simulink model "electrolizador"  (R2021a)
settings: Solver=VariableStepAuto  StartTime=0.0  StopTime=inf  RelTol=1e-3
undefined symbols (not defined in the file): magnitude
libraries: spspowerguiLib x1
settings Model: Creator=Usuario  LastModifiedBy=Usuario

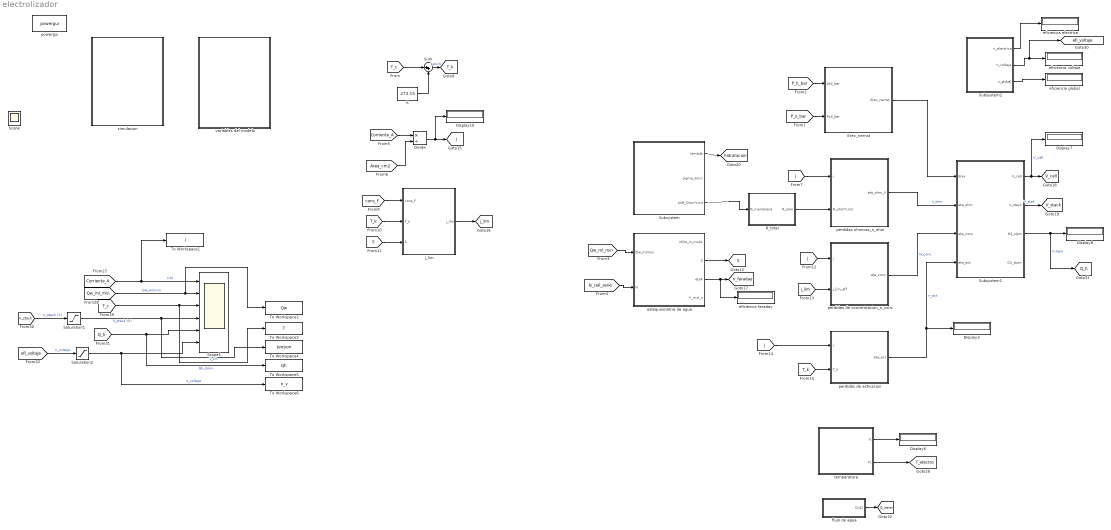
== system electrolizador ==
  Display{3,6..8,10} (5 alike) : Display
  Divide : Product  Inputs=*/
  Erev_nernst : Subsystem
  K : Constant  Value=273.15
  R_total : Subsystem
  Saturation1 : Saturate  UpperLimit=3  LowerLimit=0
  Saturation2 : Saturate  UpperLimit=1.1  LowerLimit=0
  Scope : Scope
  Scope1 : Scope  NumInputPorts=6
  Subsystem : Subsystem
  Subsystem1 : Subsystem
  Subsystem2 : Subsystem
  Sum : Sum  Inputs=|++
  To Workspace1 : ToWorkspace  VariableName=I  SaveFormat=Timeseries  SampleTime=-1
  To Workspace2 : ToWorkspace  VariableName=Qw  SaveFormat=Timeseries  SampleTime=-1
  To Workspace3 : ToWorkspace  VariableName=T  SaveFormat=Timeseries  SampleTime=-1
  To Workspace4 : ToWorkspace  VariableName=tension  SaveFormat=Timeseries  SampleTime=-1
  To Workspace5 : ToWorkspace  VariableName=Qh  SaveFormat=Timeseries  SampleTime=-1
  To Workspace6 : ToWorkspace  VariableName=n_v  SaveFormat=Timeseries  SampleTime=-1
  eficiencia electrica : Display
  eficiencia faraday : Display
  eficiencia global : Display
  eficiencia voltaje : Display
  estequiometria de agua : Subsystem
  flujo de agua : Subsystem
  j_lim : Subsystem
  perdidas de activacion : Subsystem
  perdidas de concentracion_n_conc : Subsystem
  perdidas ohmicas_n_ohm : Subsystem
  powergui : spspowerguiLib/powergui  Priority=1  SimulationMode=Discrete  SampleTime=50e-6  frequency=60  Iterations=50  frequencyindice=60  Pbase=100e6  ErrMax=1e-4  UnitsV=kV  UnitsW=MW  buscounter=0  FunctionMessages=off  echomessages=off  EnableUseOfTLC=off  CurrentSourceSwitches=off  DisableSnubberDevices=off  DisableRonSwitches=off  DisableVfSwitches=off  DisplayEquations=off  AutomaticDiscreteSolvers=off  SolverType=Tustin/Backward Euler (TBE)  Interpol=off  ExternalGateDelay=off  methode=off  Ts=100  x0status=blocks  SPID=on  SwTol=0  HookPort=off  NonlinearTolerance=1e-4  nMaxIteration=100  ContinueOnMaxIteration=off  RestoreLinks=warning  ResistiveCurrentMeasurement=off  Frange=[0:2:500]  Ylog=off  Xlog=on  ShowGrid=off  save=off  variable=ZData  structure=0  ZoomFFT=off  StartTime=0.0  cycles=1  DisplayStyle=1  fundamental=60  FreqAxis=off  MaxFrequency=1000  frequencyindicesteady=1  RmsSteady=1  display=off
  simulacion : Subsystem
  temperatura : Subsystem
  variables del modelo : Subsystem
  tag scope: Q_h=global, Q_water=global, S=global, T_electro=global, T_k=global, V_cell=global, V_stack=global, efi_voltaje=global, hidratacion=global, j=global, j_lim=global, n_faraday=global
  wires:
  K/1 -> Sum/2
  [T_c] -> Sum/1
  Sum/1 -> [T_k]  "kelvin"
  [P_o_bar] -> Erev_nernst/2(Po2_bar)
  [P_h_bar] -> Erev_nernst/1(ph2_bar)
  [Qw_ml_min] -> estequiometria de agua/1(Qw_ml/min)
  [N_cell_serie] -> estequiometria de agua/2(N)
  estequiometria de agua/2(S) -> [S]
  [Corriente_A] -> Divide/1
  [Area_cm2] -> Divide/2
  Divide/1 -> Display10/1, [j]
  Subsystem/3(ASR_Ohm*cm2) -> R_total/1(R_membrana)
  R_total/1(R_ohm) -> perdidas ohmicas_n_ohm/2(R_ohm*cm2)
  [j] -> perdidas ohmicas_n_ohm/1(j)
  [cons_F] -> j_lim/1(cons_F)
  [S] -> j_lim/3(S)
  [T_k] -> j_lim/2(T_k)
  j_lim/1(j_lim) -> [j_lim]
  [j] -> perdidas de concentracion_n_conc/1(j)
  [j_lim] -> perdidas de concentracion_n_conc/2(j_lim_eff)
  [T_k] -> perdidas de activacion/2(T_k)
  Erev_nernst/1(Erev_nernst) -> Subsystem1/1(Erev)
  perdidas ohmicas_n_ohm/1(eta_ohm_V) -> Subsystem1/2(eta_ohm)  "n_ohm"
  perdidas de concentracion_n_conc/1(eta_conc) -> Subsystem1/3(eta_conc)  "N_conc"
  estequiometria de agua/3(etaF) -> eficiencia faraday/1, [n_faraday]
  perdidas de activacion/1(eta_act) -> Subsystem1/4(eta_act), Display3/1  "n_act"
  Subsystem1/1(V_cell) -> Display7/1, [V_cell]  "V_cell"
  Subsystem1/2(V_stack) -> [V_stack]  "V_stak"
  Subsystem1/3(H2_slpm) -> [Q_h], Display8/1  "h slpm"
  Subsystem2/2(n_voltaje) -> [efi_voltaje], eficiencia voltaje/1
  Subsystem2/3(n_global) -> eficiencia global/1
  Subsystem/1(lambda) -> [hidratacion]
  [j] -> perdidas de activacion/1(j)
  temperatura/1(K) -> Display6/1
  temperatura/2(ºc) -> [T_electro]
  Subsystem2/1(n_electrica) -> eficiencia electrica/1
  [Corriente_A] -> To Workspace1/1, Scope1/1  "I(A)"
  [Qw_ml_min] -> To Workspace2/1, Scope1/2  "Qw_ml/min"
  [T_c] -> To Workspace3/1, Scope1/3  "T_Cº"
  [V_stack] -> Saturation1/1  "V_stack (V)"
  [Q_h] -> To Workspace5/1, Scope1/5  "Qh_l/min"
  [efi_voltaje] -> Saturation2/1  "n_voltaje"
  Saturation1/1 -> To Workspace4/1, Scope1/4  "V_stack (V)"
  Saturation2/1 -> To Workspace6/1, Scope1/6  "n_voltaje"
  flujo de agua/1(Out1) -> [Q_water]

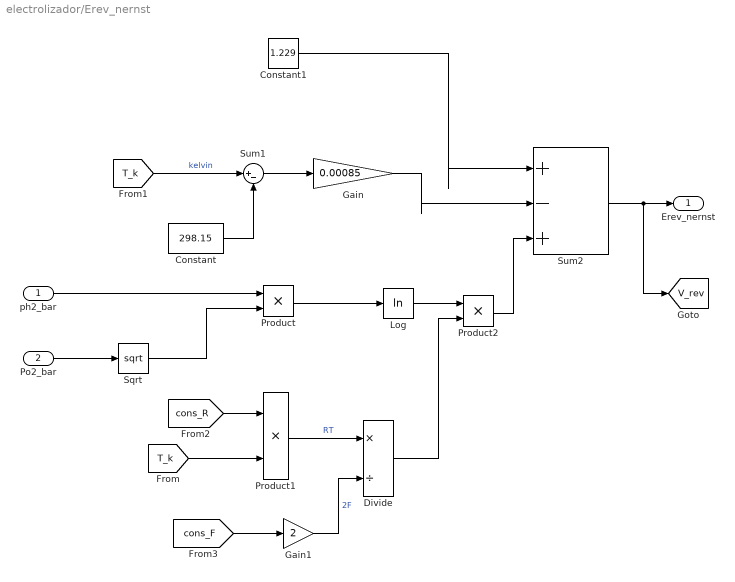
== system electrolizador/Erev_nernst ==
  ph2_bar : Inport
  Po2_bar : Inport  Port=2
  Constant : Constant  Value=298.15
  Constant1 : Constant  Value=1.229
  Divide : Product  Inputs=*/
  Gain : Gain  Gain=0.00085
  Gain1 : Gain  Gain=2
  Log : Math  Operator=log  SaturateOnIntegerOverflow=on
  Product : Product
  Product1 : Product
  Product2 : Product
  Sqrt : Sqrt  SaturateOnIntegerOverflow=on
  Sum1 : Sum  Inputs=|+-
  Sum2 : Sum  Inputs=|+-+
  Erev_nernst : Outport
  tag scope: V_rev=global
  wires:
  [T_k] -> Sum1/1  "kelvin"
  Constant/1 -> Sum1/2
  Sum1/1 -> Gain/1
  Po2_bar/1 -> Sqrt/1
  ph2_bar/1 -> Product/1
  Sqrt/1 -> Product/2
  Constant1/1 -> Sum2/1
  Gain/1 -> Sum2/2
  Product/1 -> Log/1
  [T_k] -> Product1/2
  [cons_R] -> Product1/1
  Product1/1 -> Divide/1  "RT"
  [cons_F] -> Gain1/1
  Gain1/1 -> Divide/2  "2F"
  Log/1 -> Product2/1
  Divide/1 -> Product2/2
  Product2/1 -> Sum2/3
  Sum2/1 -> [V_rev], Erev_nernst/1

== system electrolizador/R_total ==
  R_membrana : Inport
  Sum : Sum  Inputs=|++
  R_ohm : Outport
  wires:
  Sum/1 -> R_ohm/1
  R_membrana/1 -> Sum/1
  [R_contacto] -> Sum/2

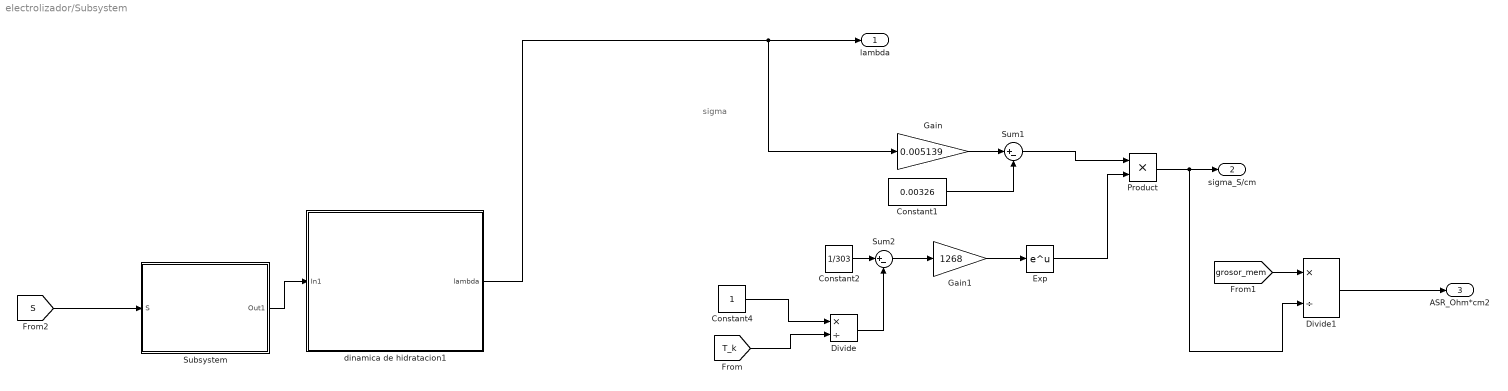
== system electrolizador/Subsystem ==
  note: sigma
  Constant1 : Constant  Value=0.00326
  Constant2 : Constant  Value=1/303
  Constant4 : Constant
  Divide : Product  Inputs=*/
  Divide1 : Product  Inputs=*/
  Exp : Math  SaturateOnIntegerOverflow=on
  Gain : Gain  Gain=0.005139
  Gain1 : Gain  Gain=1268
  Product : Product
  Subsystem : Subsystem
  Sum1 : Sum  Inputs=|+-
  Sum2 : Sum  Inputs=|+-
  dinamica de hidratacion1 : Subsystem
  lambda : Outport
  sigma_S/cm : Outport  Port=2
  ASR_Ohm*cm2 : Outport  Port=3
  wires:
  [grosor_mem] -> Divide1/1
  [T_k] -> Divide/2
  Sum2/1 -> Gain1/1
  Exp/1 -> Product/2
  Divide/1 -> Sum2/2
  Constant1/1 -> Sum1/2
  Gain/1 -> Sum1/1
  Gain1/1 -> Exp/1
  Constant4/1 -> Divide/1
  Constant2/1 -> Sum2/1
  Sum1/1 -> Product/1
  dinamica de hidratacion1/1(lambda) -> Gain/1, lambda/1
  Subsystem/1(Out1) -> dinamica de hidratacion1/1(In1)
  [S] -> Subsystem/1(S)
  Divide1/1 -> ASR_Ohm*cm2/1
  Product/1 -> Divide1/2, sigma_S/cm/1

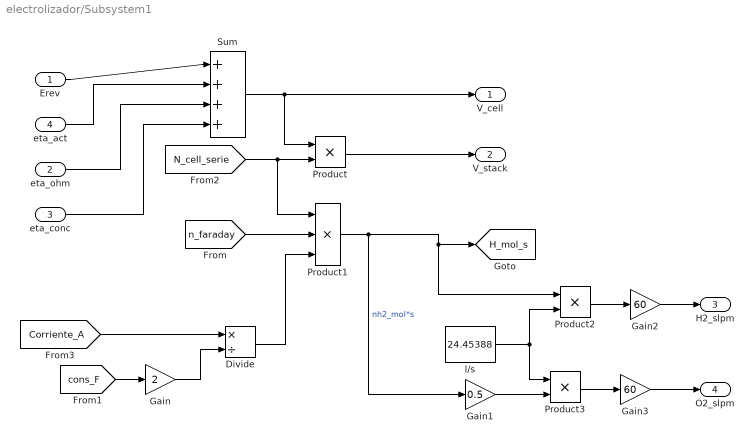
== system electrolizador/Subsystem1 ==
  Erev : Inport
  eta_ohm : Inport  Port=2
  eta_conc : Inport  Port=3
  eta_act : Inport  Port=4
  Divide : Product  Inputs=*/
  Gain : Gain  Gain=2
  Gain1 : Gain  Gain=0.5
  Gain2 : Gain  Gain=60
  Gain3 : Gain  Gain=60
  Product : Product
  Product1 : Product  Inputs=3
  Product2 : Product
  Product3 : Product
  Sum : Sum  Inputs=|++++
  l/s : Constant  Value=24.45388
  V_cell : Outport
  V_stack : Outport  Port=2
  H2_slpm : Outport  Port=3
  O2_slpm : Outport  Port=4
  tag scope: H_mol_s=global
  wires:
  Erev/1 -> Sum/1
  eta_act/1 -> Sum/2
  eta_ohm/1 -> Sum/3
  eta_conc/1 -> Sum/4
  Sum/1 -> Product/1, V_cell/1
  [N_cell_serie] -> Product1/1, Product/2
  Product/1 -> V_stack/1
  Product1/1 -> Gain1/1, [H_mol_s], Product2/1  "nh2_mol*s"
  [n_faraday] -> Product1/2
  [cons_F] -> Gain/1
  [Corriente_A] -> Divide/1
  Gain/1 -> Divide/2
  Divide/1 -> Product1/3
  Gain1/1 -> Product3/2
  l/s/1 -> Product2/2, Product3/1
  Product2/1 -> Gain2/1
  Product3/1 -> Gain3/1
  Gain2/1 -> H2_slpm/1
  Gain3/1 -> O2_slpm/1

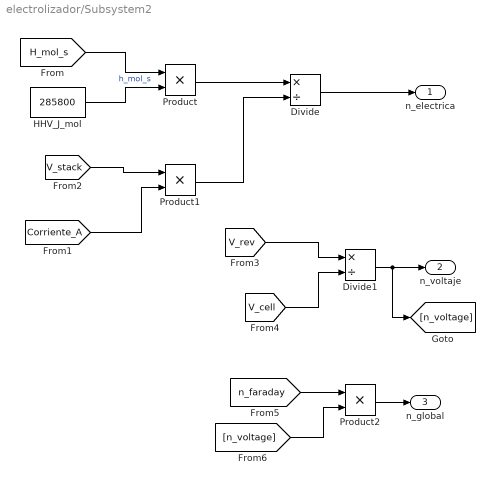
== system electrolizador/Subsystem2 ==
  Divide : Product  Inputs=*/
  Divide1 : Product  Inputs=*/
  HHV_J_mol : Constant  Value=285800
  Product : Product
  Product1 : Product
  Product2 : Product
  n_electrica : Outport
  n_voltaje : Outport  Port=2
  n_global : Outport  Port=3
  wires:
  Divide/1 -> n_electrica/1
  Product/1 -> Divide/1
  Product1/1 -> Divide/2
  [H_mol_s] -> Product/1  "h_mol_s"
  HHV_J_mol/1 -> Product/2
  [V_stack] -> Product1/1
  [Corriente_A] -> Product1/2
  Divide1/1 -> [n_voltage], n_voltaje/1
  [V_cell] -> Divide1/2
  [V_rev] -> Divide1/1
  Product2/1 -> n_global/1
  [n_faraday] -> Product2/1
  [n_voltage] -> Product2/2

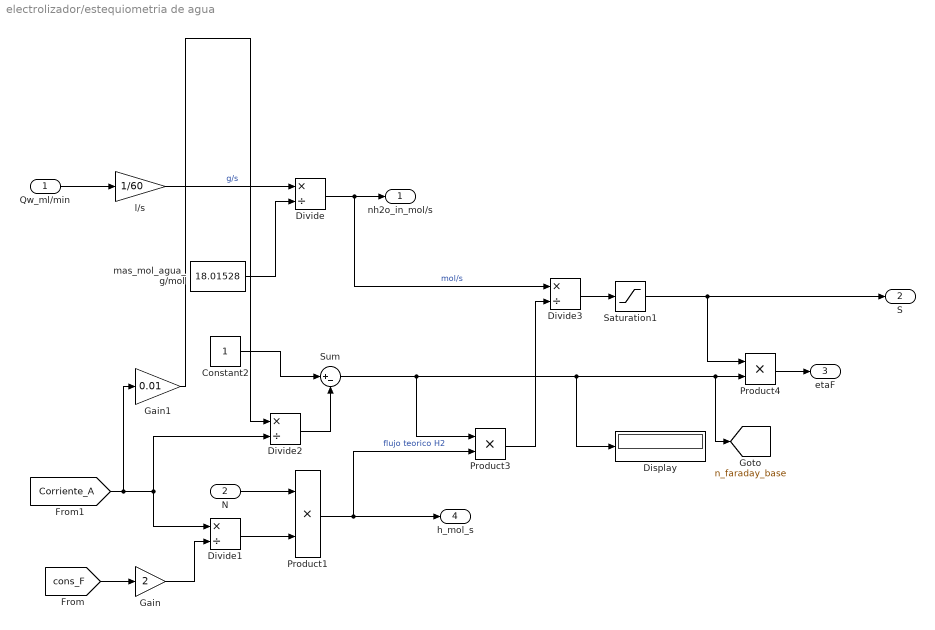
== system electrolizador/estequiometria de agua ==
  Qw_ml/min : Inport
  N : Inport  Port=2
  Constant2 : Constant
  Display : Display
  Divide{,1..3} (4 alike) : Product  Inputs=*/
  Gain : Gain  Gain=2
  Gain1 : Gain  Gain=0.01
  Product1 : Product
  Product3 : Product
  Product4 : Product
  Saturation1 : Saturate  UpperLimit=1  LowerLimit=0
  Sum : Sum  Inputs=|+-
  l/s : Gain  Gain=1/60
  mas_mol_agua_g/mol : Constant  Value=18.01528
  nh2o_in_mol/s : Outport
  S : Outport  Port=2
  etaF : Outport  Port=3
  h_mol_s : Outport  Port=4
  tag scope: n_faraday_base=global
  wires:
  l/s/1 -> Divide/1  "g/s"
  mas_mol_agua_g/mol/1 -> Divide/2
  Divide/1 -> Divide3/1, nh2o_in_mol/s/1  "mol/s"
  [cons_F] -> Gain/1
  Gain/1 -> Divide1/2
  Divide1/1 -> Product1/2
  N/1 -> Product1/1
  [Corriente_A] -> Gain1/1, Divide2/2, Divide1/1
  Constant2/1 -> Sum/1
  Divide2/1 -> Sum/2
  Sum/1 -> Product3/1, Display/1, [n_faraday_base], Product4/2
  Product1/1 -> h_mol_s/1, Product3/2  "flujo teorico H2"
  Divide3/1 -> Saturation1/1
  Product3/1 -> Divide3/2
  Product4/1 -> etaF/1
  Saturation1/1 -> Product4/1, S/1
  Qw_ml/min/1 -> l/s/1
  Gain1/1 -> Divide2/1

== system electrolizador/flujo de agua ==
  Divide : Product  Inputs=*/
  Gain : Gain  Gain=18.015
  Gain1 : Gain  Gain=60
  Gain2 : Gain  Gain=2
  Product : Product
  Out1 : Outport
  wires:
  Gain/1 -> Gain1/1
  Gain1/1 -> Out1/1
  [cons_F] -> Gain2/1
  [n_faraday_base] -> Product/1
  [Corriente_A] -> Product/2
  Product/1 -> Divide/1
  Gain2/1 -> Divide/2
  Divide/1 -> Gain/1  "mol/s"

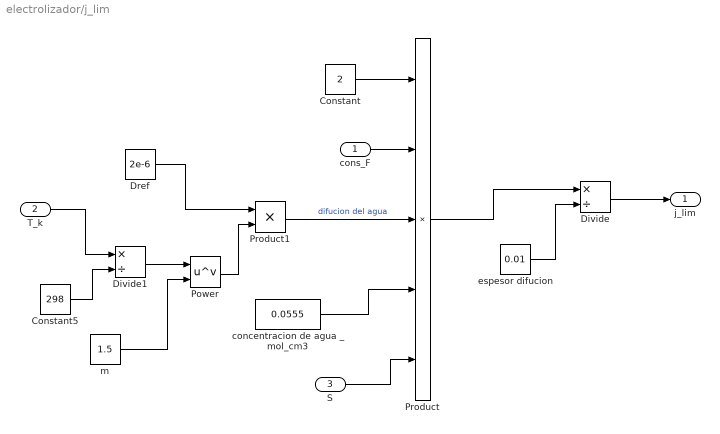
== system electrolizador/j_lim ==
  cons_F : Inport
  T_k : Inport  Port=2
  S : Inport  Port=3
  Constant : Constant  Value=2
  Constant5 : Constant  Value=298
  Divide : Product  Inputs=*/
  Divide1 : Product  Inputs=*/
  Dref : Constant  Value=2e-6
  Power : Math  Operator=pow  SaturateOnIntegerOverflow=on
  Product : Product  Inputs=5
  Product1 : Product
  concentracion de agua _mol_cm3 : Constant  Value=0.0555
  espesor difucion : Constant  Value=0.01
  m : Constant  Value=1.5
  j_lim : Outport
  wires:
  Constant/1 -> Product/1
  espesor difucion/1 -> Divide/2
  cons_F/1 -> Product/2
  Product/1 -> Divide/1
  Divide/1 -> j_lim/1
  Product1/1 -> Product/3  "difucion del agua"
  Dref/1 -> Product1/1
  Power/1 -> Product1/2
  Divide1/1 -> Power/1
  m/1 -> Power/2
  T_k/1 -> Divide1/1
  Constant5/1 -> Divide1/2
  concentracion de agua _mol_cm3/1 -> Product/4
  S/1 -> Product/5

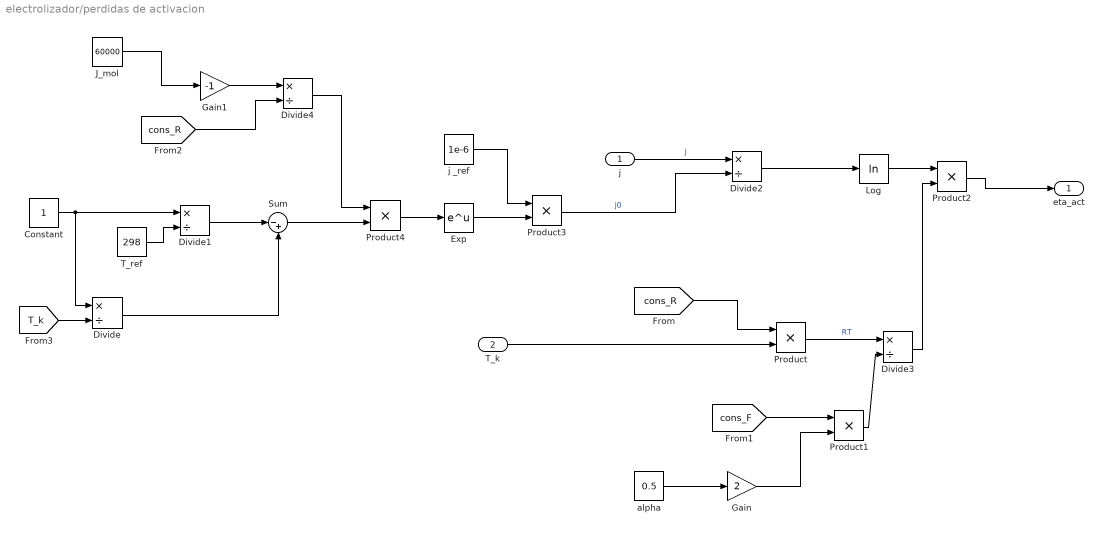
== system electrolizador/perdidas de activacion ==
  j : Inport
  T_k : Inport  Port=2
  Constant : Constant
  Divide{,1..4} (5 alike) : Product  Inputs=*/
  Exp : Math  SaturateOnIntegerOverflow=on
  Gain : Gain  Gain=2
  Gain1 : Gain  Gain=-1
  J_mol : Constant  Value=60000
  Log : Math  Operator=log  SaturateOnIntegerOverflow=on
  Product{,1..4} (5 alike) : Product
  Sum : Sum  Inputs=|-+
  T_ref : Constant  Value=298
  alpha : Constant  Value=0.5
  j _ref : Constant  Value=1e-6
  eta_act : Outport
  wires:
  j/1 -> Divide2/1  "j"
  Product3/1 -> Divide2/2  "j0"
  Divide2/1 -> Log/1
  Log/1 -> Product2/1
  [cons_R] -> Product/1
  T_k/1 -> Product/2
  [cons_F] -> Product1/1
  Product1/1 -> Divide3/2
  Product/1 -> Divide3/1  "RT"
  Divide3/1 -> Product2/2
  Product2/1 -> eta_act/1
  Gain/1 -> Product1/2
  alpha/1 -> Gain/1
  j _ref/1 -> Product3/1
  Constant/1 -> Divide/1, Divide1/1
  T_ref/1 -> Divide1/2
  Divide1/1 -> Sum/1
  Divide/1 -> Sum/2
  Sum/1 -> Product4/2
  Divide4/1 -> Product4/1
  Gain1/1 -> Divide4/1
  [cons_R] -> Divide4/2
  Product4/1 -> Exp/1
  Exp/1 -> Product3/2
  J_mol/1 -> Gain1/1
  [T_k] -> Divide/2

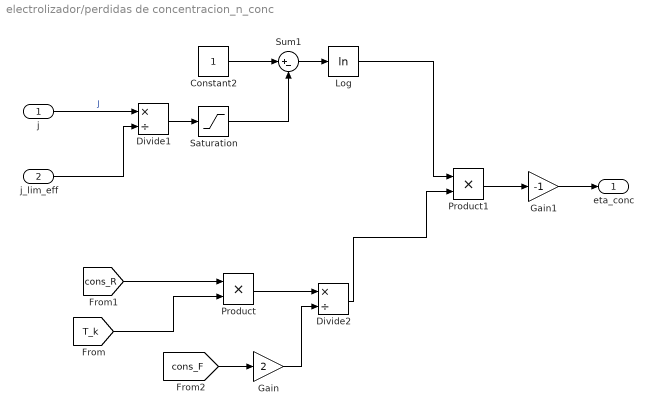
== system electrolizador/perdidas de concentracion_n_conc ==
  j : Inport
  j_lim_eff : Inport  Port=2
  Constant2 : Constant
  Divide1 : Product  Inputs=*/
  Divide2 : Product  Inputs=*/
  Gain : Gain  Gain=2
  Gain1 : Gain  Gain=-1
  Log : Math  Operator=log  SaturateOnIntegerOverflow=on
  Product : Product
  Product1 : Product
  Saturation : Saturate  UpperLimit=0.999  LowerLimit=0
  Sum1 : Sum  Inputs=|+-
  eta_conc : Outport
  wires:
  j/1 -> Divide1/1  "J"
  j_lim_eff/1 -> Divide1/2
  Divide1/1 -> Saturation/1
  Constant2/1 -> Sum1/1
  Saturation/1 -> Sum1/2
  [cons_R] -> Product/1
  [cons_F] -> Gain/1
  Product/1 -> Divide2/1
  Gain/1 -> Divide2/2
  Sum1/1 -> Log/1
  Log/1 -> Product1/1
  Product1/1 -> Gain1/1
  [T_k] -> Product/2
  Divide2/1 -> Product1/2
  Gain1/1 -> eta_conc/1

== system electrolizador/perdidas ohmicas_n_ohm ==
  j : Inport
  R_ohm*cm2 : Inport  Port=2
  Product : Product
  eta_ohm_V : Outport
  wires:
  j/1 -> Product/1  "J"
  Product/1 -> eta_ohm_V/1
  R_ohm*cm2/1 -> Product/2

== system electrolizador/simulacion ==
  Half Gauge : SemiCircularGaugeBlock  ScaleMin=20  ScaleMax=80
  Hidrogeno : DisplayBlock  LabelPosition=Hide  Format=short  Transparency=1
  Slider : SliderBlock  ScaleMax=40
  V stack : DisplayBlock  LabelPosition=Hide  Format=short  Transparency=1
  agua : DisplayBlock  LabelPosition=Hide  Format=short  Transparency=1
  corriente : DashboardScope  Ymax=40
  eficiencia electrica : LinearGaugeBlock  LabelPosition=Hide  ScaleMax=1
  eficiencia global : LinearGaugeBlock  LabelPosition=Hide  ScaleMax=1
  eficiencia voltaje : LinearGaugeBlock  LabelPosition=Hide  ScaleMax=1
  eficienia de faraday : LinearGaugeBlock  LabelPosition=Hide  ScaleMax=1
  hidratacion : DisplayBlock  LabelPosition=Hide  Format=short  Transparency=1
  inundacion : LinearGaugeBlock  LabelPosition=Hide  ScaleMax=1

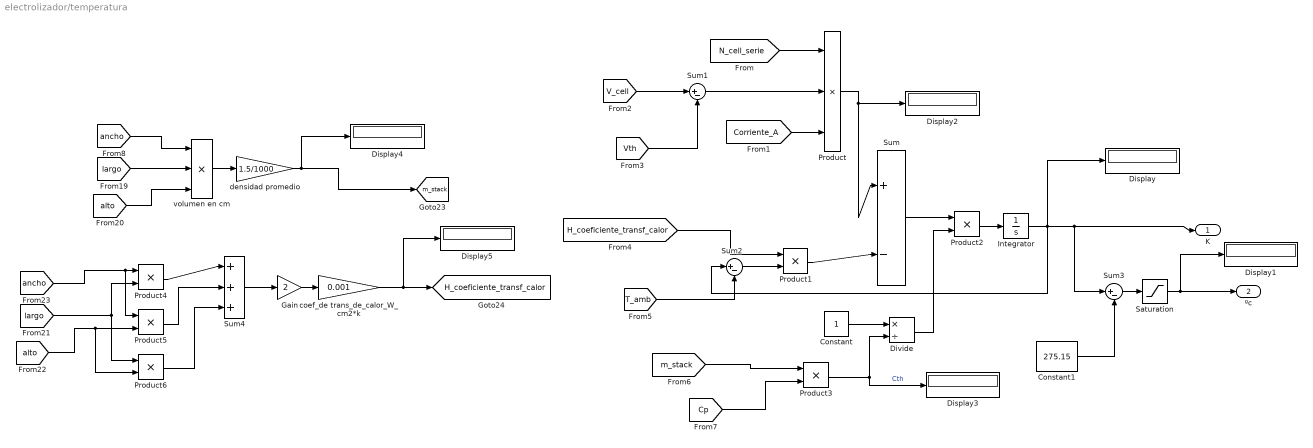
== system electrolizador/temperatura ==
  Constant : Constant
  Constant1 : Constant  Value=275.15
  Display{,1..5} (6 alike) : Display
  Divide : Product  Inputs=*/
  Gain : Gain  Gain=2
  Integrator : Integrator
  Product : Product  Inputs=3
  Product{1..6} (6 alike) : Product
  Saturation : Saturate  UpperLimit=80  LowerLimit=10
  Sum{,1..3} (4 alike) : Sum  Inputs=|+-
  Sum4 : Sum  Inputs=|+++
  coef_de trans_de_calor_W_cm2*k : Gain  Gain=0.001
  densidad promedio : Gain  Gain=1.5/1000
  volumen en cm : Product  Inputs=3
  K : Outport
  ºc : Outport  Port=2
  tag scope: H_coeficiente_transf_calor=global, m_stack=global
  wires:
  Product/1 -> Display2/1, Sum/1
  [N_cell_serie] -> Product/1
  [Corriente_A] -> Product/3
  Sum1/1 -> Product/2
  [V_cell] -> Sum1/1
  [Vth] -> Sum1/2
  Product1/1 -> Sum/2
  Sum2/1 -> Product1/2
  [H_coeficiente_transf_calor] -> Product1/1
  [T_amb] -> Sum2/2
  Sum/1 -> Product2/1
  Divide/1 -> Product2/2
  Constant/1 -> Divide/1
  Product3/1 -> Display3/1, Divide/2  "Cth"
  [Cp] -> Product3/2
  [m_stack] -> Product3/1
  Constant1/1 -> Sum3/2
  Sum3/1 -> Saturation/1
  Product2/1 -> Integrator/1
  Integrator/1 -> Sum2/1, Sum3/1, K/1, Display/1
  Saturation/1 -> Display1/1, ºc/1
  Gain/1 -> coef_de trans_de_calor_W_cm2*k/1
  volumen en cm/1 -> densidad promedio/1
  Sum4/1 -> Gain/1
  Product5/1 -> Sum4/2
  [largo] -> volumen en cm/2
  [alto] -> volumen en cm/3
  [ancho] -> volumen en cm/1
  [alto] -> Product6/2, Product5/2
  [largo] -> Product6/1, Product4/2
  [ancho] -> Product5/1, Product4/1
  coef_de trans_de_calor_W_cm2*k/1 -> Display5/1, [H_coeficiente_transf_calor]
  Product4/1 -> Sum4/1
  densidad promedio/1 -> Display4/1, [m_stack]
  Product6/1 -> Sum4/3

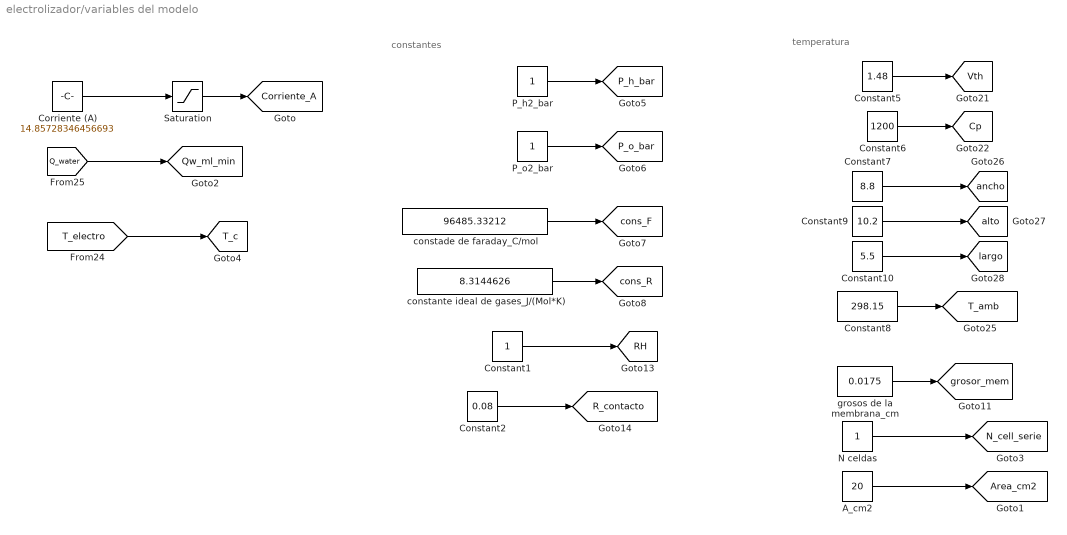
== system electrolizador/variables del modelo ==
  note: constantes
  note: temperatura
  A_cm2 : Constant  Value=20
  Constant1 : Constant
  Constant10 : Constant  Value=5.5
  Constant2 : Constant  Value=0.08
  Constant5 : Constant  Value=1.48
  Constant6 : Constant  Value=1200
  Constant7 : Constant  Value=8.8
  Constant8 : Constant  Value=298.15
  Constant9 : Constant  Value=10.2
  Corriente (A) : Constant  Value=14.85728346456693
  N celdas : Constant
  P_h2_bar : Constant
  P_o2_bar : Constant
  Saturation : Saturate  UpperLimit=40  LowerLimit=0.1
  constade de faraday_C/mol : Constant  Value=96485.33212
  constante ideal de gases_J/(Mol*K) : Constant  Value=8.3144626
  grosos de la membrana_cm : Constant  Value=0.0175
  tag scope: Area_cm2=global, Corriente_A=global, Cp=global, N_cell_serie=global, P_h_bar=global, P_o_bar=global, Qw_ml_min=global, RH=global, R_contacto=global, T_amb=global, T_c=global, Vth=global, alto=global, ancho=global, cons_F=global, cons_R=global, grosor_mem=global, largo=global
  wires:
  Constant6/1 -> [Cp]
  Constant7/1 -> [ancho]
  Constant5/1 -> [Vth]
  Constant9/1 -> [alto]
  Constant10/1 -> [largo]
  Constant8/1 -> [T_amb]
  [Q_water] -> [Qw_ml_min]
  Corriente (A)/1 -> Saturation/1
  [T_electro] -> [T_c]
  Saturation/1 -> [Corriente_A]
  N celdas/1 -> [N_cell_serie]
  A_cm2/1 -> [Area_cm2]
  grosos de la membrana_cm/1 -> [grosor_mem]
  Constant1/1 -> [RH]
  P_h2_bar/1 -> [P_h_bar]
  P_o2_bar/1 -> [P_o_bar]
  constade de faraday_C/mol/1 -> [cons_F]
  constante ideal de gases_J/(Mol*K)/1 -> [cons_R]
  Constant2/1 -> [R_contacto]

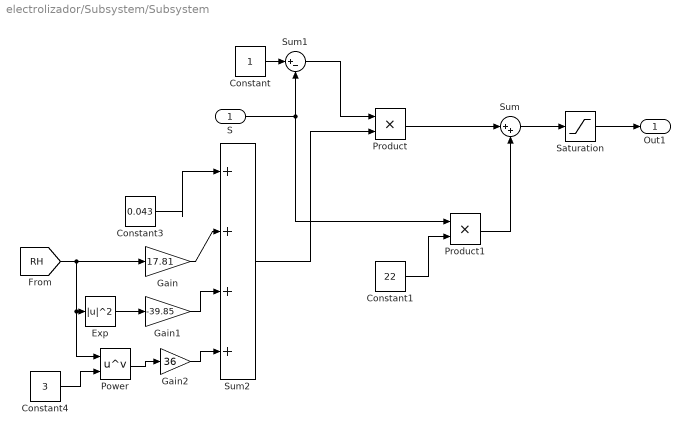
== system electrolizador/Subsystem/Subsystem ==
  S : Inport
  Constant : Constant
  Constant1 : Constant  Value=22
  Constant3 : Constant  Value=0.043
  Constant4 : Constant  Value=3
  Exp : Math  Operator=magnitude^2  SaturateOnIntegerOverflow=on
  Gain : Gain  Gain=17.81
  Gain1 : Gain  Gain=-39.85
  Gain2 : Gain  Gain=36
  Power : Math  Operator=pow  SaturateOnIntegerOverflow=on
  Product : Product
  Product1 : Product
  Saturation : Saturate  UpperLimit=22  LowerLimit=0
  Sum : Sum  Inputs=|++
  Sum1 : Sum  Inputs=|+-
  Sum2 : Sum  Inputs=|++++
  Out1 : Outport
  wires:
  Product/1 -> Sum/1
  Product1/1 -> Sum/2
  Constant1/1 -> Product1/2
  Constant/1 -> Sum1/1
  Sum1/1 -> Product/1
  Sum2/1 -> Product/2
  S/1 -> Product1/1, Sum1/2
  Sum/1 -> Saturation/1
  Constant3/1 -> Sum2/1
  Gain1/1 -> Sum2/3
  Gain2/1 -> Sum2/4
  Gain/1 -> Sum2/2
  Exp/1 -> Gain1/1
  [RH] -> Power/1, Exp/1, Gain/1
  Power/1 -> Gain2/1
  Constant4/1 -> Power/2
  Saturation/1 -> Out1/1

== system electrolizador/Subsystem/dinamica de hidratacion1 ==
  In1 : Inport
  Gain : Gain  Gain=1/0.5
  Integrator : Integrator
  Product1 : Product
  Product2 : Product
  Saturation : Saturate  UpperLimit=22  LowerLimit=0
  Sign : Signum
  Sum5 : Sum  Inputs=|+-
  Sum6 : Sum  Inputs=|++
  k_back : Constant
  k_drag : Constant  Value=0.2
  lambda : Outport
  wires:
  k_back/1 -> Product1/1
  Sign/1 -> Product2/1
  Product1/1 -> Gain/1
  k_drag/1 -> Product2/2
  Product2/1 -> Sum6/2
  Sum5/1 -> Product1/2
  Sum6/1 -> Integrator/1
  In1/1 -> Sum5/1
  Integrator/1 -> Sum5/2, Saturation/1
  Gain/1 -> Sum6/1
  [Corriente_A] -> Sign/1
  Saturation/1 -> lambda/1
